simulink model "ALTITUDE_DYNAMICS_MODEL"  (R2024b)
settings: Solver=VariableStepAuto  StartTime=0.0  StopTime=60  RelTol=1e-3
values from neighbouring files (symbols this model uses):
  A_alt_aug = [A_alt, zeros(size(A_alt,1),1); -C_alt, 0]    [ALTITUDE_DYNAMICS.m]
  B_alt_aug = [B_alt; 0]    [ALTITUDE_DYNAMICS.m]
  C_alt_aug = [C_alt 0]    [ALTITUDE_DYNAMICS.m]
  D_alt_aug = D_alt    [ALTITUDE_DYNAMICS.m]
  q1_alt = 10    [ALTITUDE_DYNAMICS.m]
  q2_alt = 1    [ALTITUDE_DYNAMICS.m]
  q3_alt = 5    [ALTITUDE_DYNAMICS.m]
  q4_alt = 15    [ALTITUDE_DYNAMICS.m]
  R_alt = 1    [ALTITUDE_DYNAMICS.m]
settings Model: Creator=hazza  LastModifiedBy=hazza

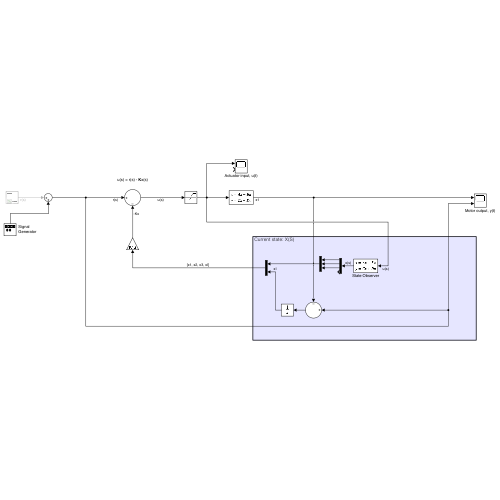
[thumbnail: Simulink's stored preview of the top-level diagram]
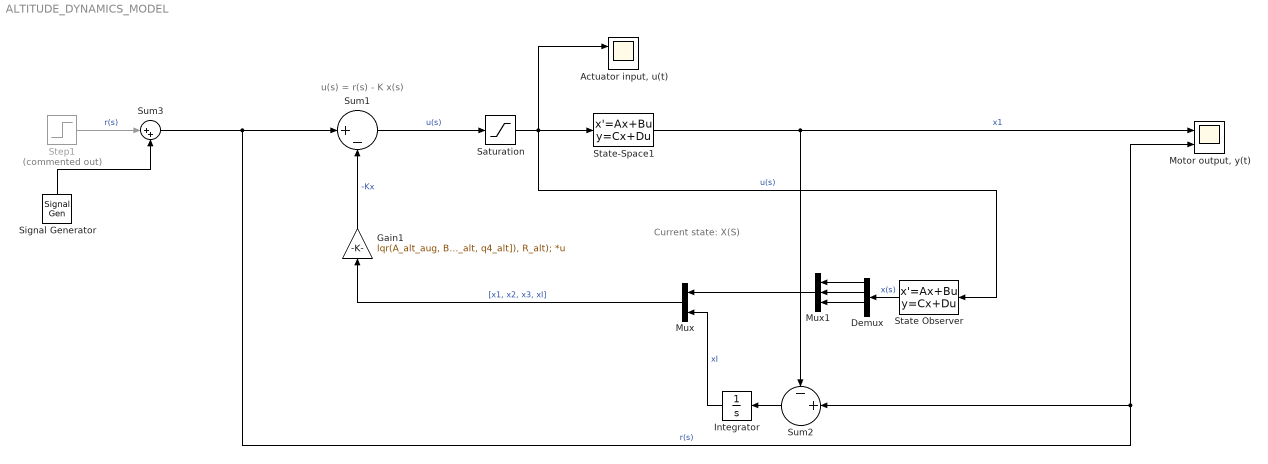
== system ALTITUDE_DYNAMICS_MODEL ==
  note: Current state: X(S)
  note: u(s) = r(s) - K x(s)
  "Actuator input, u(t)" : Scope  NumInputPorts=2
  Demux : Demux
  Gain1 : Gain  Gain=lqr(A_alt_aug, B_alt_aug, diag([q1_alt, q2_alt, q3_alt, q4_alt]), R_alt);  Multiplication=Matrix(K*u)
  Integrator : Integrator
  "Motor output, y(t)" : Scope  NumInputPorts=2
  Mux : Mux  Inputs=2
  Mux1 : Mux  Inputs=3
  Saturation : Saturate  UpperLimit=95  LowerLimit=-55  ZeroCross=off
  Signal Generator : SignalGenerator  Amplitude=-1  Frequency=1/5  Units=rad/sec
  State Observer : StateSpace  A=A_alt_aug  B=B_alt_aug  C=eye(4)  D=zeros(4,1)  InitialCondition=[0, 0, 0, 0]
  State-Space1 : StateSpace  A=A_alt_aug  B=B_alt_aug  C=C_alt_aug  D=D_alt_aug  InitialCondition=[0, 0, 0,0]
  Step1 : Step  Commented=on  Time=10  Before=1200  After=800  SampleTime=0
  Sum1 : Sum  Inputs=|+-
  Sum2 : Sum  Inputs=-+|
  Sum3 : Sum  Inputs=|++
  wires:
  Gain1/1 -> Sum1/2  "-Kx"
  State-Space1/1 -> Sum2/1, "Motor output, y(t)"/1  "x1"
  Sum3/1 -> Sum1/1, "Motor output, y(t)"/2, Sum2/2  "r(s)"
  Sum1/1 -> Saturation/1  "u(s)"
  Saturation/1 -> State Observer/1, "Actuator input, u(t)"/1, State-Space1/1  "u(s)"
  Step1/1 -> Sum3/1  "r(s)"
  Signal Generator/1 -> Sum3/2
  Sum2/1 -> Integrator/1
  Integrator/1 -> Mux/2  "xI"
  Mux/1 -> Gain1/1  "[x1, x2, x3, xI]"
  State Observer/1 -> Demux/1  "x(s)"
  Demux/1 -> Mux1/1
  Demux/2 -> Mux1/2
  Demux/3 -> Mux1/3
  Mux1/1 -> Mux/1
